simulink model "PLL_Analog"  (R2024a)
settings: Solver=ode45  StartTime=0.0  StopTime=1  RelTol=1e-6  EnableMultiTasking=on
InitFcn:
  | addpath Simulaciones_PLL
  | run parametros_PLL_a.m
values from neighbouring files (symbols this model uses):
  Cf = 1e-6    (= 1e-06)    [parametros_PLL_a.m]
  Kvco = (2*N*fi)/VDD    (= 320)    [parametros_PLL_a.m]
  R1 = 10e3    (= 10000)    [parametros_PLL_a.m]
  R2 = 200e3    (= 200000)    [parametros_PLL_a.m]
  Ts = 1e-3    (= 0.001)    [PLL_dig_coeff.m]    (also in parametros_PLL_a.m = 5e-05)
  VDD = 10    [parametros_PLL_a.m]
libraries: msbPllFoundation x1
settings Model: Creator=nicolas  LastModifiedBy=svanico
settings SolverCC: AlgebraicLoopSolver=TrustRegion  SolverResetMethod=Robust
settings DataIOCC: LimitDataPoints=on  SaveFormat=Array  SignalLoggingSaveFormat=ModelDataLogs  ReturnWorkspaceOutputs=off
settings OptimizationCC: ExpressionDepthLimit=2147483647  LifeSpan=inf
settings DebuggingCC: UnderspecifiedInitializationDetection=Classic  MergeDetectMultiDrivingBlocksExec=none  SolverPrmCheckMsg=warning  FcnCallInpInsideContextMsg=warning  UnconnectedInputMsg=warning  UnconnectedOutputMsg=warning  UnconnectedLineMsg=warning  StateNameClashWarn=warning  SFUnexpectedBacktrackingDiag=warning  SFNoUnconditionalDefaultTransitionDiag=warning  SFExecutionAtInitializationDiag=none  ArithmeticOperatorsInVariantConditions=warning
settings HardwareCC: ProdBitPerPointer=32  ProdBitPerSizeT=32  ProdBitPerPtrDiffT=32  ProdLargestAtomicFloat=None  ProdIntDivRoundTo=Undefined  ProdEndianess=Unspecified  ProdWordSize=32  ProdHWDeviceType=32-bit Generic
settings ModelReferenceCC: PropagateSignalLabelsOutOfModel=off
settings SFSimCC: SimUseLocalCustomCode=off  CustomCodeUndefinedFunction=UseInterfaceOnly
settings RTWCC: RTWUseLocalCustomCode=off  GPUComputeCapability=3.5
settings CodeAppCC: StateflowObjectComments=on
settings GRTTargetCC: TargetLangStandard=C89/C90 (ANSI)  CombineOutputUpdateFcns=off  GRTInterface=on
settings ConfigComp: CovMetricSettings=dw  CovSaveCumulativeToWorkspaceVar=on  CovSaveSingleToWorkspaceVar=on  CovExternalEMLEnable=off

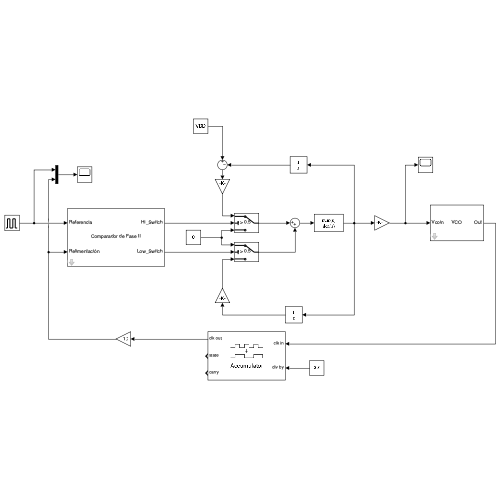
[thumbnail: Simulink's stored preview of the top-level diagram]
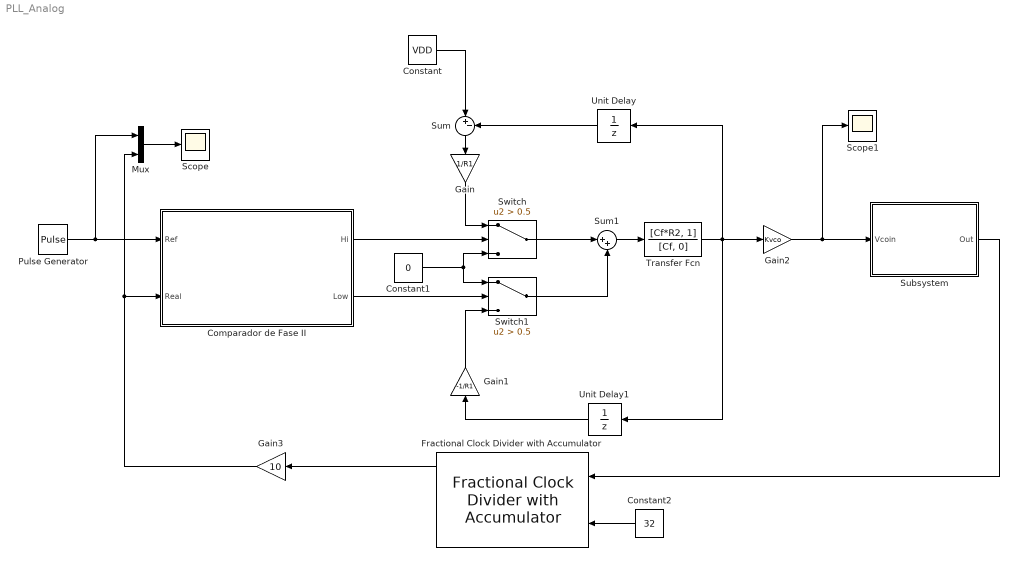
== system PLL_Analog ==
  Comparador de Fase II : Subsystem  mask{Ts=Ts}
      mask Display:
      | disp('Comparador de Fase II')
      | port_label('input',1,'Referencia')
      | port_label('input',2,'Relimentación')
      | port_label('output',1,'Hi_Switch')
      | port_label('output',2,'Low_Switch')
  Constant : Constant  Value=VDD
  Constant1 : Constant  Value=0
  Constant2 : Constant  Value=32
  Fractional Clock Divider with Accumulator : msbPllFoundation/Fractional Clock Divider with Accumulator  ExtraBuffer=on  NBuffer=1000
  Gain : Gain  Gain=1/R1
  Gain1 : Gain  Gain=-1/R1
  Gain2 : Gain  Gain=Kvco
  Gain3 : Gain  Gain=10
  Mux : Mux  Inputs=2
  Pulse Generator : DiscretePulseGenerator  PulseType=Time based  Amplitude=10  Period=1/50  PulseWidth=50
  Scope : Scope
  Scope1 : Scope
  Subsystem : Subsystem  mask{Ts=Ts}
      mask Display:
      | disp('VCO')
      | port_label('input',1,'Vcoin')
      | port_label('output',1,'Out')
  Sum : Sum  Inputs=|+-
  Sum1 : Sum  Inputs=|++
  Switch : Switch  Criteria=u2 > Threshold  Threshold=0.5  SaturateOnIntegerOverflow=off  InputSameDT=off
  Switch1 : Switch  Criteria=u2 > Threshold  Threshold=0.5  SaturateOnIntegerOverflow=off  InputSameDT=off
  Transfer Fcn : TransferFcn  Numerator=[Cf*R2, 1]  Denominator=[Cf, 0]
  Unit Delay : UnitDelay  SampleTime=-1  HasFrameUpgradeWarning=on
  Unit Delay1 : UnitDelay  SampleTime=-1  HasFrameUpgradeWarning=on
  wires:
  Pulse Generator/1 -> Mux/1, Comparador de Fase II/1(Ref)
  Sum1/1 -> Transfer Fcn/1
  Constant/1 -> Sum/1
  Sum/1 -> Gain/1
  Gain/1 -> Switch/1
  Comparador de Fase II/1(Hi) -> Switch/2
  Constant1/1 -> Switch1/1, Switch/3
  Comparador de Fase II/2(Low) -> Switch1/2
  Switch/1 -> Sum1/1
  Switch1/1 -> Sum1/2
  Gain2/1 -> Scope1/1, Subsystem/1(Vcoin)
  Subsystem/1(Out) -> Fractional Clock Divider with Accumulator/1
  Constant2/1 -> Fractional Clock Divider with Accumulator/2
  Fractional Clock Divider with Accumulator/1 -> Gain3/1
  Mux/1 -> Scope/1
  Gain3/1 -> Mux/2, Comparador de Fase II/2(Real)
  Gain1/1 -> Switch1/3
  Transfer Fcn/1 -> Unit Delay/1, Unit Delay1/1, Gain2/1
  Unit Delay/1 -> Sum/2
  Unit Delay1/1 -> Gain1/1

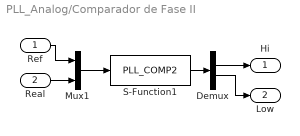
== system PLL_Analog/Comparador de Fase II ==
  Ref : Inport
  Real : Inport  Port=2
  Demux : Demux
  Mux1 : Mux  Inputs=2
  S-Function1 : S-Function  FunctionName=PLL_COMP2  Parameters=Ts  SFunctionDeploymentMode=off  EnableBusSupport=off
  Hi : Outport
  Low : Outport  Port=2
  wires:
  Mux1/1 -> S-Function1/1
  S-Function1/1 -> Demux/1
  Ref/1 -> Mux1/1
  Demux/2 -> Hi/1
  Demux/3 -> Low/1
  Real/1 -> Mux1/2

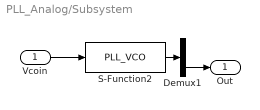
== system PLL_Analog/Subsystem ==
  Vcoin : Inport
  Demux1 : Demux  Outputs=2
  S-Function2 : S-Function  FunctionName=PLL_VCO  Parameters=Ts  SFunctionDeploymentMode=off  EnableBusSupport=off
  Out : Outport
  wires:
  S-Function2/1 -> Demux1/1
  Vcoin/1 -> S-Function2/1
  Demux1/2 -> Out/1
